simulink model "GbxFr_Unit"  (R2020b)
settings: configuration reference "gen_config" (kept outside this file)
libraries: simulink_extras x1
settings Model: DataDictionary=Hybrid_vehicle.sldd  SimulationMode=accelerator  OrderedModelArguments=off  Creator=Georg  LastModifiedBy=jy
settings ConfigSetRef: SourceName=gen_config

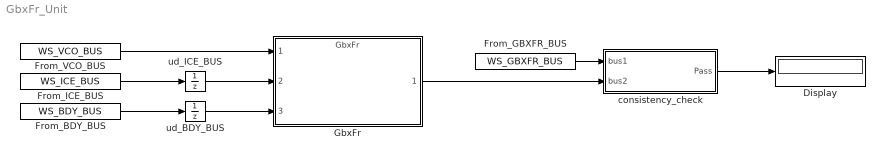
== system GbxFr_Unit ==
  Display : Display
  From_BDY_BUS : FromWorkspace  VariableName=WS_BDY_BUS  OutDataTypeStr=Bus: BDY_BUS  SampleTime=-1  Interpolate=off  OutputAfterFinalValue=Holding final value
  From_GBXFR_BUS : FromWorkspace  VariableName=WS_GBXFR_BUS  OutDataTypeStr=Bus: GBXFR_BUS  SampleTime=-1  Interpolate=off  OutputAfterFinalValue=Holding final value
  From_ICE_BUS : FromWorkspace  VariableName=WS_ICE_BUS  OutDataTypeStr=Bus: ICE_BUS  SampleTime=-1  Interpolate=off  OutputAfterFinalValue=Holding final value
  From_VCO_BUS : FromWorkspace  VariableName=WS_VCO_BUS  OutDataTypeStr=Bus: VCO_BUS  SampleTime=-1  Interpolate=off  OutputAfterFinalValue=Holding final value
  GbxFr : ModelReference  ModelNameDialog=GbxFr  SimulationMode=Normal  ModelReferenceVersion=2.27
  consistency_check : Subsystem
  ud_BDY_BUS : UnitDelay  SampleTime=-1  HasFrameUpgradeWarning=on
  ud_ICE_BUS : UnitDelay  SampleTime=-1  HasFrameUpgradeWarning=on
  wires:
  From_VCO_BUS/1 -> GbxFr/1
  From_ICE_BUS/1 -> ud_ICE_BUS/1
  ud_ICE_BUS/1 -> GbxFr/2
  From_BDY_BUS/1 -> ud_BDY_BUS/1
  ud_BDY_BUS/1 -> GbxFr/3
  From_GBXFR_BUS/1 -> consistency_check/1(bus1)
  GbxFr/1 -> consistency_check/2(bus2)
  consistency_check/1(Pass) -> Display/1

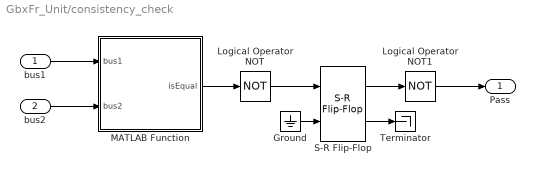
== system GbxFr_Unit/consistency_check ==
  bus1 : Inport
  bus2 : Inport  Port=2
  Ground : Ground
  Logical Operator NOT : Logic  Operator=NOT  AllPortsSameDT=off  OutDataTypeStr=boolean
  Logical Operator NOT1 : Logic  Operator=NOT  AllPortsSameDT=off  OutDataTypeStr=boolean
  MATLAB Function : MATLAB Function  TreatAsAtomicUnit=on
  S-R Flip-Flop : simulink_extras/Flip Flops/S-R Flip-Flop  initial_condition=0
  Terminator : Terminator
  Pass : Outport
  wires:
  bus1/1 -> MATLAB Function/1(bus1)
  bus2/1 -> MATLAB Function/2(bus2)
  MATLAB Function/1(isEqual) -> Logical Operator NOT/1
  Logical Operator NOT/1 -> S-R Flip-Flop/1
  Ground/1 -> S-R Flip-Flop/2
  S-R Flip-Flop/2 -> Terminator/1
  S-R Flip-Flop/1 -> Logical Operator NOT1/1
  Logical Operator NOT1/1 -> Pass/1

== matlab function GbxFr_Unit/consistency_check/MATLAB Function ==
  data: bus1 input; isEqual output; bus2 input
function isEqual = fcn(bus1, bus2)
isEqual = isequal(bus1, bus2);
